simulink model "Car_Modelling"  (R2022a)
settings: Solver=VariableStepAuto  StartTime=0.0  StopTime=3.543  RelTol=1e-3
settings Model: Creator=amitkm  LastModifiedBy=amitkm

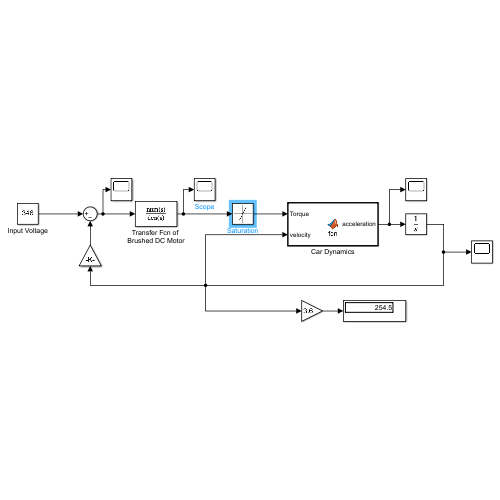
[thumbnail: Simulink's stored preview of the top-level diagram]
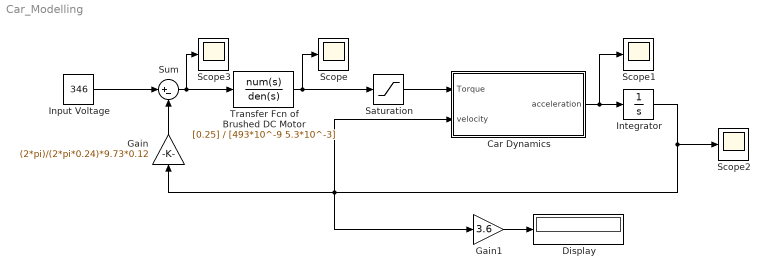
== system Car_Modelling ==
  Car Dynamics : MATLAB Function  TreatAsAtomicUnit=on
  Display : Display
  Gain : Gain  Gain=(2*pi)/(2*pi*0.24)*9.73*0.12
  Gain1 : Gain  Gain=3.6
  Input Voltage : Constant  Value=346
  Integrator : Integrator
  Saturation : Saturate  UpperLimit=601  LowerLimit=0
  Scope{,1..3} (4 alike) : Scope
  Sum : Sum  Inputs=|+-
  Transfer Fcn of Brushed DC Motor : TransferFcn  Numerator=[0.25]  Denominator=[493*10^-9 5.3*10^-3]
  wires:
  Input Voltage/1 -> Sum/1
  Gain/1 -> Sum/2
  Sum/1 -> Scope3/1, Transfer Fcn of Brushed DC Motor/1
  Transfer Fcn of Brushed DC Motor/1 -> Scope/1, Saturation/1
  Integrator/1 -> Scope2/1, Gain1/1, Gain/1, Car Dynamics/2(velocity)
  Car Dynamics/1(acceleration) -> Scope1/1, Integrator/1
  Gain1/1 -> Display/1
  Saturation/1 -> Car Dynamics/1(Torque)

== matlab function Car_Modelling/Car Dynamics ==
  data: Torque input; acceleration output; velocity input
function acceleration = fcn(Torque, velocity)
acceleration=(40.5*Torque*0.6-413-0.3381*velocity^2)/2108;
